simulink model "lab12"  (R2017a)
settings: Solver=VariableStepAuto  StartTime=0.0  StopTime=10.0  RelTol=1e-3
InitFcn:
  | f
values from neighbouring files (symbols this model uses):
  a = 2.75    [f.m]
  b = 1.3    [f.m]
  x = -7.85    [f.m]
settings Model: Creator=Peter  LastModifiedBy=Peter

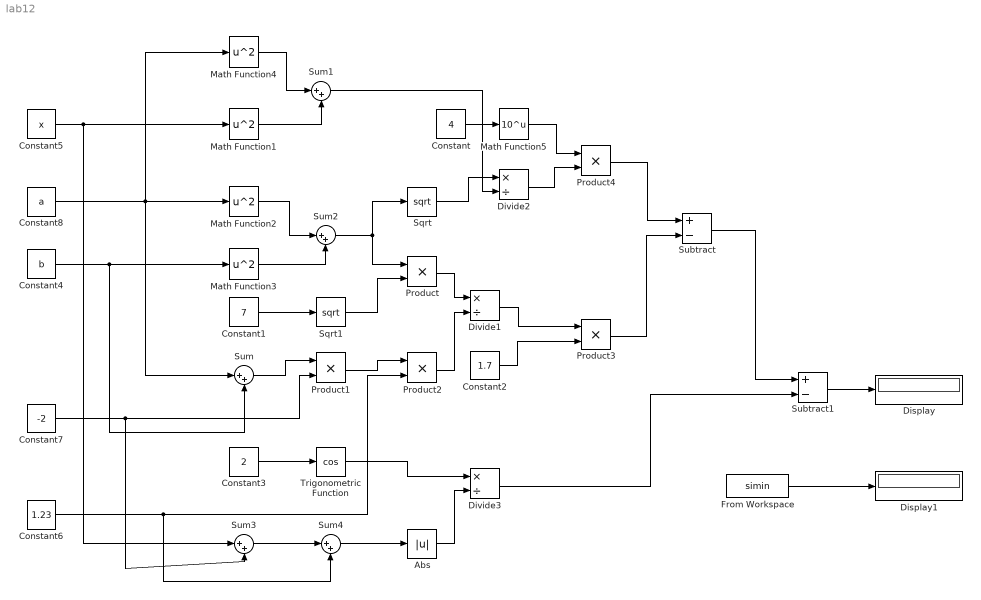
== system lab12 ==
  Abs : Abs
  Constant : Constant  Value=4
  Constant1 : Constant  Value=7
  Constant2 : Constant  Value=1.7
  Constant3 : Constant  Value=2
  Constant4 : Constant  Value=b
  Constant5 : Constant  Value=x
  Constant6 : Constant  Value=1.23
  Constant7 : Constant  Value=-2
  Constant8 : Constant  Value=a
  Display : Display
  Display1 : Display
  Divide1 : Product  Inputs=*/
  Divide2 : Product  Inputs=*/
  Divide3 : Product  Inputs=*/
  From Workspace : FromWorkspace  VariableName=simin  Interpolate=off  OutputAfterFinalValue=Holding final value
  Math Function{1..4} (4 alike) : Math  Operator=square  SaturateOnIntegerOverflow=on
  Math Function5 : Math  Operator=10^u  SaturateOnIntegerOverflow=on
  Product{,1..4} (5 alike) : Product
  Sqrt : Sqrt  SaturateOnIntegerOverflow=on
  Sqrt1 : Sqrt  SaturateOnIntegerOverflow=on
  Subtract : Sum  Inputs=+-
  Subtract1 : Sum  Inputs=+-
  Sum{,1..4} (5 alike) : Sum  Inputs=|++
  Trigonometric Function : Trigonometry  Operator=cos
  wires:
  Math Function2/1 -> Sum2/1
  Math Function3/1 -> Sum2/2
  Sum2/1 -> Product/1, Sqrt/1
  Sqrt1/1 -> Product/2
  Constant1/1 -> Sqrt1/1
  Product/1 -> Divide1/1
  Product2/1 -> Divide1/2
  Product1/1 -> Product2/1
  Sum/1 -> Product1/1
  Divide1/1 -> Product3/1
  Constant2/1 -> Product3/2
  Math Function4/1 -> Sum1/1
  Math Function1/1 -> Sum1/2
  Divide2/1 -> Product4/2
  Constant/1 -> Math Function5/1
  Math Function5/1 -> Product4/1
  Constant3/1 -> Trigonometric Function/1
  Product4/1 -> Subtract/1
  Product3/1 -> Subtract/2
  Sum4/1 -> Abs/1
  Sum3/1 -> Sum4/1
  Abs/1 -> Divide3/2
  Trigonometric Function/1 -> Divide3/1
  Subtract/1 -> Subtract1/1
  Divide3/1 -> Subtract1/2
  Subtract1/1 -> Display/1
  Constant8/1 -> Sum/1, Math Function4/1, Math Function2/1
  Constant4/1 -> Sum/2, Math Function3/1
  Sqrt/1 -> Divide2/1
  Sum1/1 -> Divide2/2
  Constant5/1 -> Sum3/1, Math Function1/1
  Constant7/1 -> Sum3/2, Product1/2
  Constant6/1 -> Sum4/2, Product2/2
  From Workspace/1 -> Display1/1
